simulink library "NSA_DEVS_DIGITAL_FLIPFLOP"  (R2022b)
settings: Solver=VariableStepAuto  StartTime=0.0  StopTime=10.0  RelTol=1e-3
libraries: NSA_DEVS_DIGITAL_LOGIC x8, $bdroot x2
settings Model: Creator=david  LastModifiedBy=david

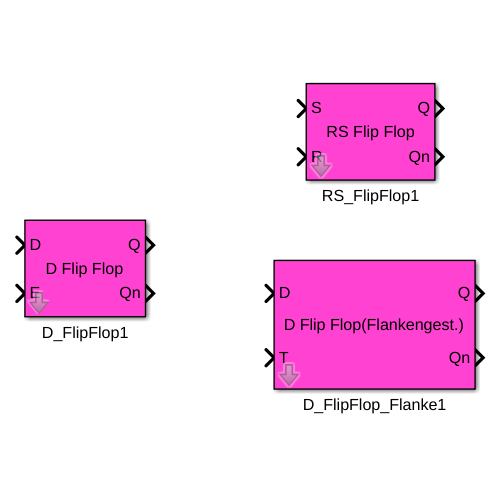
[thumbnail: Simulink's stored preview of the top-level diagram]
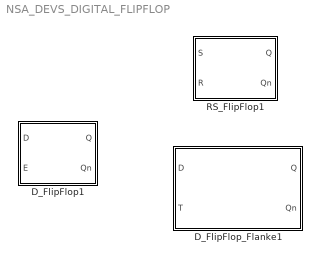
== system NSA_DEVS_DIGITAL_FLIPFLOP ==
  D_FlipFlop1 : Subsystem  mask{tau=[0,1], debug=0, constructor='D_FlipFlop("name", tau, debug)'}
      mask Display:
      | disp("D Flip Flop");
      | 
      | port_label('input', 1, 'D');
      | port_label('input', 2, 'E');
      | port_label('output', 1, 'Q');
      | port_label('output', 2, 'Qn');
  D_FlipFlop_Flanke1 : Subsystem  mask{tau=[0,1], debug=0, constructor='D_FlipFlop_Flanke("name", tau, debug)'}
      mask Display:
      | disp("D Flip Flop(Flankengest.)");
      | 
      | port_label('input', 1, 'D');
      | port_label('input', 2, 'T');
      | port_label('output', 1, 'Q');
      | port_label('output', 2, 'Qn');
  RS_FlipFlop1 : Subsystem  mask{tau=[0,1], debug=0, constructor='RS_FlipFlop("name", tau, debug)'}
      mask Display:
      | disp("RS Flip Flop");
      | 
      | port_label('input', 1, 'S');
      | port_label('input', 2, 'R');
      | port_label('output', 1, 'Q');
      | port_label('output', 2, 'Qn');

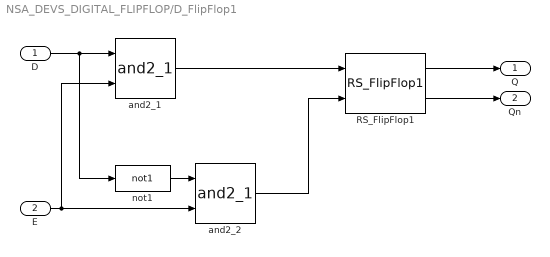
== system NSA_DEVS_DIGITAL_FLIPFLOP/D_FlipFlop1 ==
  D : Inport
  E : Inport  Port=2
  RS_FlipFlop1 : $bdroot/RS_FlipFlop1  tau=tau  debug=debug  constructor="'RS_FlipFlop(\"name\", tau, debug)'"
      settings: LibrarySourceBlock=NSA_DEVS_LIB/RS_FlipFlop1
  and2_1 : NSA_DEVS_DIGITAL_LOGIC/and2_1  tau=tau  debug=debug  constructor="'and2(\"name\", tau, debug)'"
      settings: LibrarySourceBlock=NSA_DEVS_LIB/and2_1  SourceProductName=NSA_DEVS
  and2_2 : NSA_DEVS_DIGITAL_LOGIC/and2_1  tau=tau  debug=debug  constructor="'and2(\"name\", tau, debug)'"
      settings: LibrarySourceBlock=NSA_DEVS_LIB/and2_1  SourceProductName=NSA_DEVS
  not1 : NSA_DEVS_DIGITAL_LOGIC/not1  tau=tau  debug=debug  constructor="'not(\"name\",tau,debug)'"
      settings: LibrarySourceBlock=NSA_DEVS_LIB/not1  SourceProductName=NSA_DEVS
  Q : Outport
  Qn : Outport  Port=2
  wires:
  RS_FlipFlop1/2 -> Qn/1
  RS_FlipFlop1/1 -> Q/1
  D/1 -> not1/1, and2_1/1
  E/1 -> and2_2/2, and2_1/2
  and2_1/1 -> RS_FlipFlop1/1
  and2_2/1 -> RS_FlipFlop1/2
  not1/1 -> and2_2/1

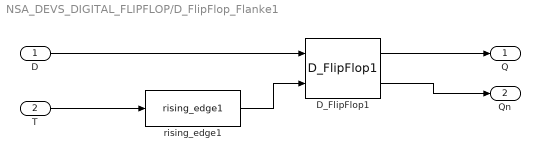
== system NSA_DEVS_DIGITAL_FLIPFLOP/D_FlipFlop_Flanke1 ==
  D : Inport
  T : Inport  Port=2
  D_FlipFlop1 : $bdroot/D_FlipFlop1  tau=tau  debug=debug  constructor="'RS_FlipFlop(\"name\", tau, debug)'"
      settings: LibrarySourceBlock=NSA_DEVS_LIB/D_FlipFlop1
  rising_edge1 : NSA_DEVS_DIGITAL_LOGIC/rising_edge1  tau=tau  debug=debug  constructor="'Rising_Edge(\"name\", tau, debug)'"
      settings: LibrarySourceBlock=NSA_DEVS_LIB/rising_edge1  SourceProductName=NSA_DEVS
  Q : Outport
  Qn : Outport  Port=2
  wires:
  D_FlipFlop1/1 -> Q/1
  D_FlipFlop1/2 -> Qn/1
  D/1 -> D_FlipFlop1/1
  rising_edge1/1 -> D_FlipFlop1/2
  T/1 -> rising_edge1/1

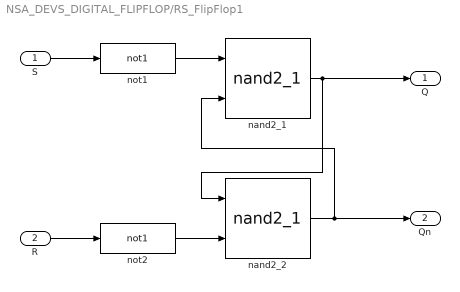
== system NSA_DEVS_DIGITAL_FLIPFLOP/RS_FlipFlop1 ==
  S : Inport
  R : Inport  Port=2
  nand2_1 : NSA_DEVS_DIGITAL_LOGIC/nand2_1  tau=tau  debug=debug  constructor="'nand2(\"name\", tau, debug)'"
      settings: LibrarySourceBlock=NSA_DEVS_LIB/nand2_1  SourceProductName=NSA_DEVS
  nand2_2 : NSA_DEVS_DIGITAL_LOGIC/nand2_1  tau=2*tau  debug=debug  constructor="'nand2(\"name\", tau, debug)'"
      settings: LibrarySourceBlock=NSA_DEVS_LIB/nand2_1  SourceProductName=NSA_DEVS
  not1 : NSA_DEVS_DIGITAL_LOGIC/not1  tau=tau  debug=debug  constructor="'not(\"name\",tau,debug)'"
      settings: LibrarySourceBlock=NSA_DEVS_LIB/not1  SourceProductName=NSA_DEVS
  not2 : NSA_DEVS_DIGITAL_LOGIC/not1  tau=tau  debug=debug  constructor="'not(\"name\",tau,debug)'"
      settings: LibrarySourceBlock=NSA_DEVS_LIB/not1  SourceProductName=NSA_DEVS
  Q : Outport
  Qn : Outport  Port=2
  wires:
  nand2_2/1 -> Qn/1, nand2_1/2
  nand2_1/1 -> nand2_2/1, Q/1
  not1/1 -> nand2_1/1
  not2/1 -> nand2_2/2
  S/1 -> not1/1
  R/1 -> not2/1
